simulink model "mtv1_with_slosh"  (R2014b)
settings: Solver=ode4  SolverMode=SingleTasking  StartTime=0.0  StopTime=sim_stop_time  FixedStep=sim_time_step_size  RelTol=1e-3
PreLoadFcn:
  | nimbus_bus_all;
  | mtv_bus_all;
undefined symbols (not defined in the file or in its folder): csc_egt_egc_thruster, csc_egt_egc_thruster_lib, csc_eom_six_dof_integration_fwdeuler, csc_eom_six_dof_integration_lib, csc_rigid_body_dynamics, csc_rigid_body_dynamics_lib, csc_sim_mtv_simulation, csc_sim_mtv_simulation_lib, csc_thl_thrusters_mtv, csc_thl_thrusters_mtv_lib, csci_gsse_mtv, csci_gsse_mtv_lib, csu_rrk_rotational_kinematics, csu_rrk_rotational_kinematics_lib, csu_rtk_translational_kinematics, csu_rtk_translational_kinematics_lib, csu_tpl_thruster_propellant_mtv, csu_tpl_thruster_propellant_mtv_lib, egt_feed_pressure, egt_g_times_isp, egt_pc_to_thrust_offset, egt_pc_to_thrust_slope, ini_epoch_seconds, ini_landed_flag, ini_thrust_to_weight_takeoff_limit, mpl_gn2_mass_initial, mpl_htp_mass_initial, sim_time_step_size, swm_num_switches, tpl_coarse_acs_thrust_to_isp, tpl_egc_chamber_pressure_to_thrust, tpl_egc_throttle_to_mdot_gain, tpl_egc_throttle_to_thrust, tpl_egc_throttle_to_thrust_gain
libraries: util_common_lib x13, util_info_lib x10, simulink x8, csu_spv_simulated_press_valves_lib x4, util_quat_lib x3, util_event_lib x2, util_frame_rotation_lib x2, csci_fsw_mtv_lib x1, csc_gnd_sta_lib x1, telem_conversion_lib x1, util_thruster_lib x1, csc_enf_environmental_forces_mtv_lib x1
(part 2 of 2)

== system mtv1_with_slosh/csci_gsse_mtv/csc_sim_mtv_simulation/csc_rigid_body_dynamics/csc_eom_six_dof_integration_fwdeuler/csu_rrk_rotational_kinematics_a/quaternion_propagator ==
  initial_q : Inport
  omega : Inport  Port=2
  reset : Inport  Port=3
  Constant1 : Constant  Value=0
  Discrete-Time Integrator1 : DiscreteIntegrator  ExternalReset=rising  InitialConditionSource=external  SampleTime=sim_time_step_size
  Library Information : util_info_lib/Library Information  owner='NONE'
  Sum1 : Sum  Inputs=|++
  quaternion_derivative : util_quat_lib/quaternion_derivative  SystemSampleTime=-1
  unit_vector : util_common_lib/unit_vector  SystemSampleTime=-1
  quat : Outport
  wires:
  omega/1 -> quaternion_derivative/1
  unit_vector/1 -> quaternion_derivative/2, quat/1
  quaternion_derivative/1 -> Discrete-Time Integrator1/1
  Sum1/1 -> unit_vector/1
  reset/1 -> Discrete-Time Integrator1/2
  initial_q/1 -> Sum1/1
  Discrete-Time Integrator1/1 -> Sum1/2
  Constant1/1 -> Discrete-Time Integrator1/3
